simulink model "test_mdl_gw"  (R2018a)
settings: Solver=VariableStepAuto  StartTime=0.0  StopTime=10.0  RelTol=1e-3
(part 1 of 2)
settings Model: Creator=HIL105  LastModifiedBy=HIL105

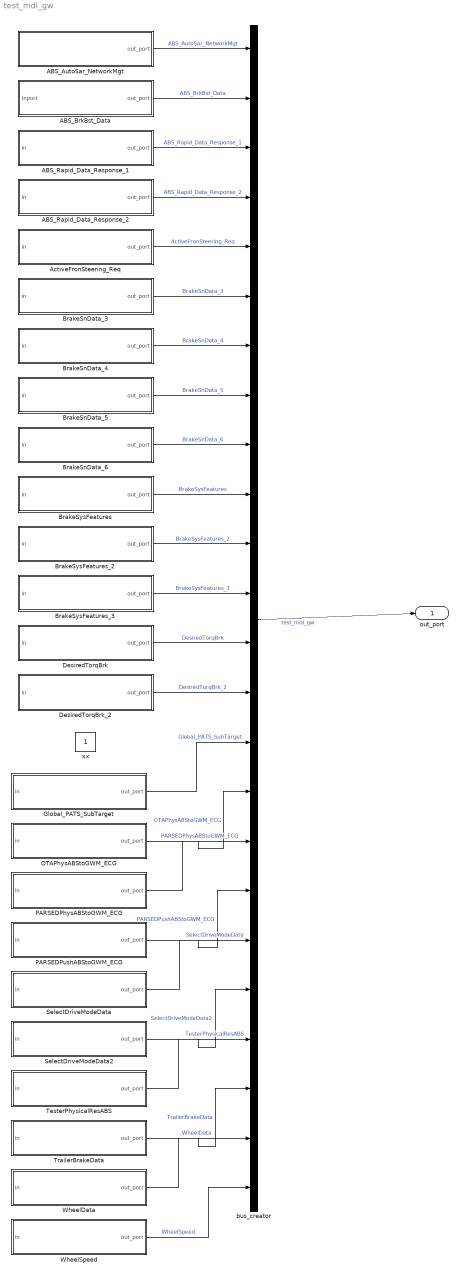
== system test_mdl_gw ==
  ABS_AutoSar_NetworkMgt : Subsystem
  ABS_BrkBst_Data : Subsystem
  ABS_Rapid_Data_Response_1 : Subsystem
  ABS_Rapid_Data_Response_2 : Subsystem
  ActiveFronSteering_Req : Subsystem
  BrakeSnData_3 : Subsystem
  BrakeSnData_4 : Subsystem
  BrakeSnData_5 : Subsystem
  BrakeSnData_6 : Subsystem
  BrakeSysFeatures : Subsystem
  BrakeSysFeatures_2 : Subsystem
  BrakeSysFeatures_3 : Subsystem
  DesiredTorqBrk : Subsystem
  DesiredTorqBrk_2 : Subsystem
  Global_PATS_SubTarget : Subsystem
  OTAPhysABStoGWM_ECG : Subsystem
  PARSEDPhysABStoGWM_ECG : Subsystem
  PARSEDPushABStoGWM_ECG : Subsystem
  SelectDriveModeData : Subsystem
  SelectDriveModeData2 : Subsystem
  TesterPhysicalResABS : Subsystem
  TrailerBrakeData : Subsystem
  WheelData : Subsystem
  WheelSpeed : Subsystem
  bus_creator : BusCreator  Inputs=24
  xx : Constant
  out_port : Outport
  wires:
  bus_creator/1 -> out_port/1  "test_mdl_gw"
  ABS_AutoSar_NetworkMgt/1(out_port) -> bus_creator/1  "ABS_AutoSar_NetworkMgt"
  ABS_BrkBst_Data/1(out_port) -> bus_creator/2  "ABS_BrkBst_Data"
  ABS_Rapid_Data_Response_1/1(out_port) -> bus_creator/3  "ABS_Rapid_Data_Response_1"
  ABS_Rapid_Data_Response_2/1(out_port) -> bus_creator/4  "ABS_Rapid_Data_Response_2"
  ActiveFronSteering_Req/1(out_port) -> bus_creator/5  "ActiveFronSteering_Req"
  BrakeSnData_3/1(out_port) -> bus_creator/6  "BrakeSnData_3"
  BrakeSnData_4/1(out_port) -> bus_creator/7  "BrakeSnData_4"
  BrakeSnData_5/1(out_port) -> bus_creator/8  "BrakeSnData_5"
  BrakeSnData_6/1(out_port) -> bus_creator/9  "BrakeSnData_6"
  BrakeSysFeatures/1(out_port) -> bus_creator/10  "BrakeSysFeatures"
  BrakeSysFeatures_2/1(out_port) -> bus_creator/11  "BrakeSysFeatures_2"
  BrakeSysFeatures_3/1(out_port) -> bus_creator/12  "BrakeSysFeatures_3"
  DesiredTorqBrk/1(out_port) -> bus_creator/13  "DesiredTorqBrk"
  DesiredTorqBrk_2/1(out_port) -> bus_creator/14  "DesiredTorqBrk_2"
  Global_PATS_SubTarget/1(out_port) -> bus_creator/15  "Global_PATS_SubTarget"
  OTAPhysABStoGWM_ECG/1(out_port) -> bus_creator/16  "OTAPhysABStoGWM_ECG"
  PARSEDPhysABStoGWM_ECG/1(out_port) -> bus_creator/17  "PARSEDPhysABStoGWM_ECG"
  PARSEDPushABStoGWM_ECG/1(out_port) -> bus_creator/18  "PARSEDPushABStoGWM_ECG"
  SelectDriveModeData/1(out_port) -> bus_creator/19  "SelectDriveModeData"
  SelectDriveModeData2/1(out_port) -> bus_creator/20  "SelectDriveModeData2"
  TesterPhysicalResABS/1(out_port) -> bus_creator/21  "TesterPhysicalResABS"
  TrailerBrakeData/1(out_port) -> bus_creator/22  "TrailerBrakeData"
  WheelData/1(out_port) -> bus_creator/23  "WheelData"
  WheelSpeed/1(out_port) -> bus_creator/24  "WheelSpeed"

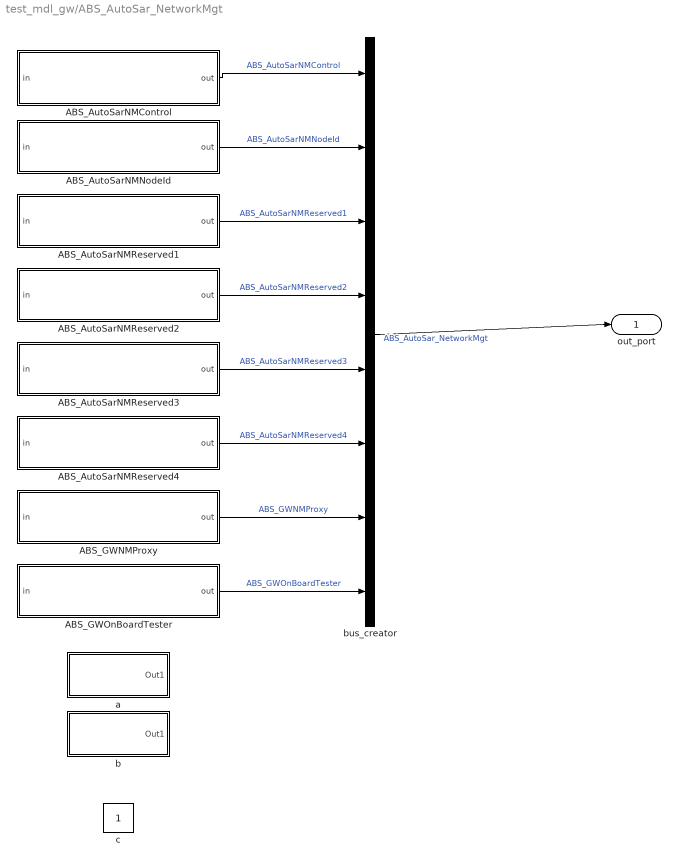
== system test_mdl_gw/ABS_AutoSar_NetworkMgt ==
  ABS_AutoSarNMControl : Subsystem
  ABS_AutoSarNMNodeId : Subsystem
  ABS_AutoSarNMReserved1 : Subsystem
  ABS_AutoSarNMReserved2 : Subsystem
  ABS_AutoSarNMReserved3 : Subsystem
  ABS_AutoSarNMReserved4 : Subsystem
  ABS_GWNMProxy : Subsystem
  ABS_GWOnBoardTester : Subsystem
  a : Subsystem
  b : Subsystem
  bus_creator : BusCreator  Inputs=8
  c : Constant
  out_port : Outport
  wires:
  bus_creator/1 -> out_port/1  "ABS_AutoSar_NetworkMgt"
  ABS_AutoSarNMControl/1(out) -> bus_creator/1  "ABS_AutoSarNMControl"
  ABS_AutoSarNMNodeId/1(out) -> bus_creator/2  "ABS_AutoSarNMNodeId"
  ABS_AutoSarNMReserved1/1(out) -> bus_creator/3  "ABS_AutoSarNMReserved1"
  ABS_AutoSarNMReserved2/1(out) -> bus_creator/4  "ABS_AutoSarNMReserved2"
  ABS_AutoSarNMReserved3/1(out) -> bus_creator/5  "ABS_AutoSarNMReserved3"
  ABS_AutoSarNMReserved4/1(out) -> bus_creator/6  "ABS_AutoSarNMReserved4"
  ABS_GWNMProxy/1(out) -> bus_creator/7  "ABS_GWNMProxy"
  ABS_GWOnBoardTester/1(out) -> bus_creator/8  "ABS_GWOnBoardTester"

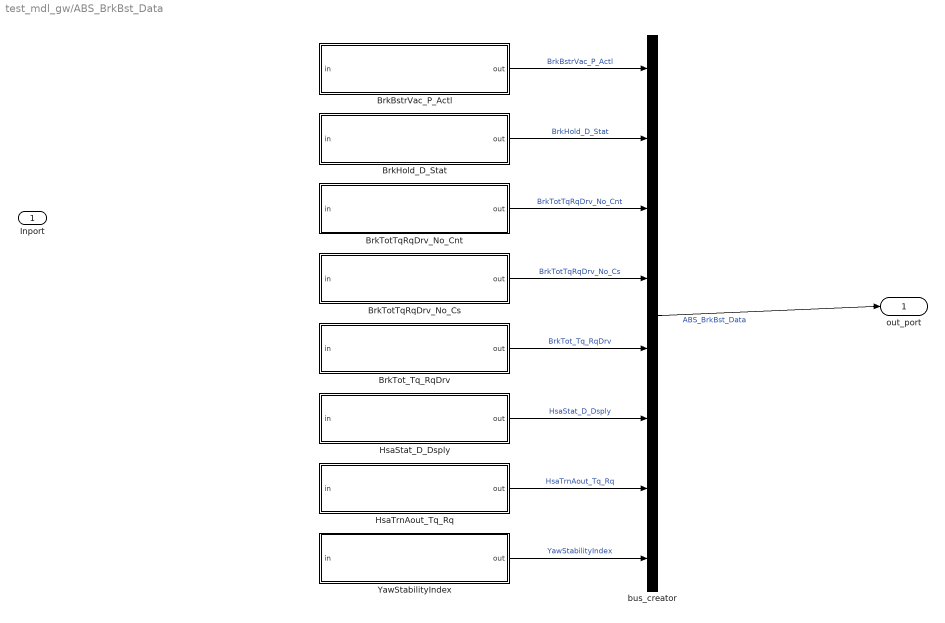
== system test_mdl_gw/ABS_BrkBst_Data ==
  Inport : Inport
  BrkBstrVac_P_Actl : Subsystem
  BrkHold_D_Stat : Subsystem
  BrkTotTqRqDrv_No_Cnt : Subsystem
  BrkTotTqRqDrv_No_Cs : Subsystem
  BrkTot_Tq_RqDrv : Subsystem
  HsaStat_D_Dsply : Subsystem
  HsaTrnAout_Tq_Rq : Subsystem
  YawStabilityIndex : Subsystem
  bus_creator : BusCreator  Inputs=8
  out_port : Outport
  wires:
  bus_creator/1 -> out_port/1  "ABS_BrkBst_Data"
  BrkBstrVac_P_Actl/1(out) -> bus_creator/1  "BrkBstrVac_P_Actl"
  BrkHold_D_Stat/1(out) -> bus_creator/2  "BrkHold_D_Stat"
  BrkTotTqRqDrv_No_Cnt/1(out) -> bus_creator/3  "BrkTotTqRqDrv_No_Cnt"
  BrkTotTqRqDrv_No_Cs/1(out) -> bus_creator/4  "BrkTotTqRqDrv_No_Cs"
  BrkTot_Tq_RqDrv/1(out) -> bus_creator/5  "BrkTot_Tq_RqDrv"
  HsaStat_D_Dsply/1(out) -> bus_creator/6  "HsaStat_D_Dsply"
  HsaTrnAout_Tq_Rq/1(out) -> bus_creator/7  "HsaTrnAout_Tq_Rq"
  YawStabilityIndex/1(out) -> bus_creator/8  "YawStabilityIndex"

== system test_mdl_gw/ABS_Rapid_Data_Response_1 ==
  in : Inport
  UUDTABSResponse1 : Subsystem
  bus_creator : BusCreator  Inputs=1
  bus_selector : BusSelector  OutputSignals=UUDTABSResponse1
  out_port : Outport
  wires:
  bus_creator/1 -> out_port/1  "ABS_Rapid_Data_Response_1"
  UUDTABSResponse1/1(out) -> bus_creator/1  "UUDTABSResponse1"
  bus_selector/1 -> UUDTABSResponse1/1(in)  "<UUDTABSResponse1>"
  in/1 -> bus_selector/1

== system test_mdl_gw/ABS_Rapid_Data_Response_2 ==
  in : Inport
  UUDTABSResponse2 : Subsystem
  bus_creator : BusCreator  Inputs=1
  bus_selector : BusSelector  OutputSignals=UUDTABSResponse2
  out_port : Outport
  wires:
  bus_creator/1 -> out_port/1  "ABS_Rapid_Data_Response_2"
  UUDTABSResponse2/1(out) -> bus_creator/1  "UUDTABSResponse2"
  bus_selector/1 -> UUDTABSResponse2/1(in)  "<UUDTABSResponse2>"
  in/1 -> bus_selector/1

== system test_mdl_gw/ActiveFronSteering_Req ==
  in : Inport
  SteWhlBrkAnRq_No_Cnt : Subsystem
  SteWhlBrkAnRq_No_Cs : Subsystem
  SteWhlBrkOffst_An_Rq : Subsystem
  bus_creator : BusCreator  Inputs=3
  bus_selector : BusSelector  OutputSignals=SteWhlBrkAnRq_No_Cnt,SteWhlBrkAnRq_No_Cs,SteWhlBrkOffst_An_Rq
  out_port : Outport
  wires:
  bus_creator/1 -> out_port/1  "ActiveFronSteering_Req"
  SteWhlBrkAnRq_No_Cnt/1(out) -> bus_creator/1  "SteWhlBrkAnRq_No_Cnt"
  SteWhlBrkAnRq_No_Cs/1(out) -> bus_creator/2  "SteWhlBrkAnRq_No_Cs"
  SteWhlBrkOffst_An_Rq/1(out) -> bus_creator/3  "SteWhlBrkOffst_An_Rq"
  bus_selector/1 -> SteWhlBrkAnRq_No_Cnt/1(in)  "<SteWhlBrkAnRq_No_Cnt>"
  bus_selector/2 -> SteWhlBrkAnRq_No_Cs/1(in)  "<SteWhlBrkAnRq_No_Cs>"
  bus_selector/3 -> SteWhlBrkOffst_An_Rq/1(in)  "<SteWhlBrkOffst_An_Rq>"
  in/1 -> bus_selector/1

== system test_mdl_gw/BrakeSnData_3 ==
  in : Inport
  VehLatComp_A_Actl : Subsystem
  VehLongComp_A_Actl : Subsystem
  VehOverGnd_V_Est : Subsystem
  VehTrvlDir_D_Stat : Subsystem
  VehYawComp_W_Actl : Subsystem
  bus_creator : BusCreator  Inputs=5
  bus_selector : BusSelector  OutputSignals=VehLatComp_A_Actl,VehLongComp_A_Actl,VehOverGnd_V_Est,VehTrvlDir_D_Stat,VehYawComp_W_Actl
  out_port : Outport
  wires:
  bus_creator/1 -> out_port/1  "BrakeSnData_3"
  VehLatComp_A_Actl/1(out) -> bus_creator/1  "VehLatComp_A_Actl"
  VehLongComp_A_Actl/1(out) -> bus_creator/2  "VehLongComp_A_Actl"
  VehOverGnd_V_Est/1(out) -> bus_creator/3  "VehOverGnd_V_Est"
  VehTrvlDir_D_Stat/1(out) -> bus_creator/4  "VehTrvlDir_D_Stat"
  VehYawComp_W_Actl/1(out) -> bus_creator/5  "VehYawComp_W_Actl"
  bus_selector/1 -> VehLatComp_A_Actl/1(in)  "<VehLatComp_A_Actl>"
  bus_selector/2 -> VehLongComp_A_Actl/1(in)  "<VehLongComp_A_Actl>"
  bus_selector/3 -> VehOverGnd_V_Est/1(in)  "<VehOverGnd_V_Est>"
  bus_selector/4 -> VehTrvlDir_D_Stat/1(in)  "<VehTrvlDir_D_Stat>"
  bus_selector/5 -> VehYawComp_W_Actl/1(in)  "<VehYawComp_W_Actl>"
  in/1 -> bus_selector/1

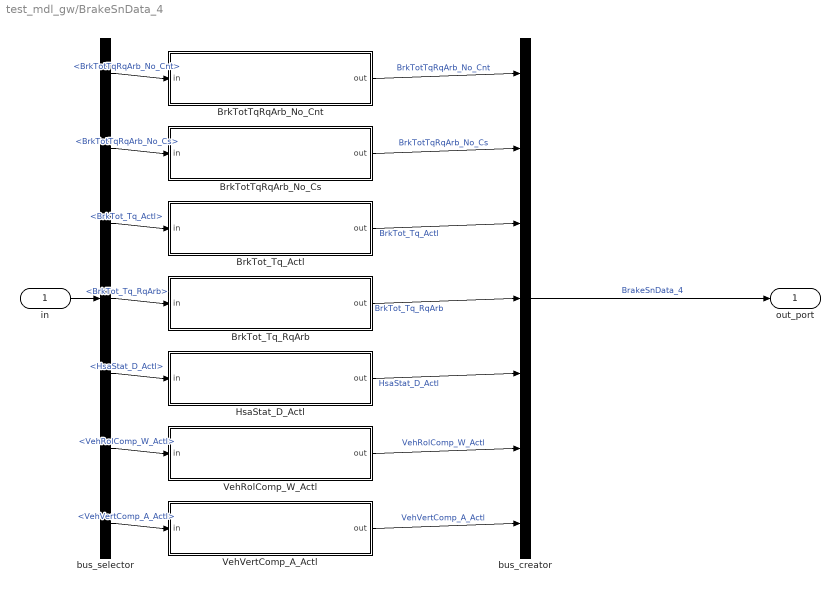
== system test_mdl_gw/BrakeSnData_4 ==
  in : Inport
  BrkTotTqRqArb_No_Cnt : Subsystem
  BrkTotTqRqArb_No_Cs : Subsystem
  BrkTot_Tq_Actl : Subsystem
  BrkTot_Tq_RqArb : Subsystem
  HsaStat_D_Actl : Subsystem
  VehRolComp_W_Actl : Subsystem
  VehVertComp_A_Actl : Subsystem
  bus_creator : BusCreator  Inputs=7
  bus_selector : BusSelector  OutputSignals=BrkTotTqRqArb_No_Cnt,BrkTotTqRqArb_No_Cs,BrkTot_Tq_Actl,BrkTot_Tq_RqArb,HsaStat_D_Actl,VehRolComp_W_Actl,VehVertComp_A_Actl
  out_port : Outport
  wires:
  bus_creator/1 -> out_port/1  "BrakeSnData_4"
  BrkTotTqRqArb_No_Cnt/1(out) -> bus_creator/1  "BrkTotTqRqArb_No_Cnt"
  BrkTotTqRqArb_No_Cs/1(out) -> bus_creator/2  "BrkTotTqRqArb_No_Cs"
  BrkTot_Tq_Actl/1(out) -> bus_creator/3  "BrkTot_Tq_Actl"
  BrkTot_Tq_RqArb/1(out) -> bus_creator/4  "BrkTot_Tq_RqArb"
  HsaStat_D_Actl/1(out) -> bus_creator/5  "HsaStat_D_Actl"
  VehRolComp_W_Actl/1(out) -> bus_creator/6  "VehRolComp_W_Actl"
  VehVertComp_A_Actl/1(out) -> bus_creator/7  "VehVertComp_A_Actl"
  bus_selector/1 -> BrkTotTqRqArb_No_Cnt/1(in)  "<BrkTotTqRqArb_No_Cnt>"
  bus_selector/2 -> BrkTotTqRqArb_No_Cs/1(in)  "<BrkTotTqRqArb_No_Cs>"
  bus_selector/3 -> BrkTot_Tq_Actl/1(in)  "<BrkTot_Tq_Actl>"
  bus_selector/4 -> BrkTot_Tq_RqArb/1(in)  "<BrkTot_Tq_RqArb>"
  bus_selector/5 -> HsaStat_D_Actl/1(in)  "<HsaStat_D_Actl>"
  bus_selector/6 -> VehRolComp_W_Actl/1(in)  "<VehRolComp_W_Actl>"
  bus_selector/7 -> VehVertComp_A_Actl/1(in)  "<VehVertComp_A_Actl>"
  in/1 -> bus_selector/1

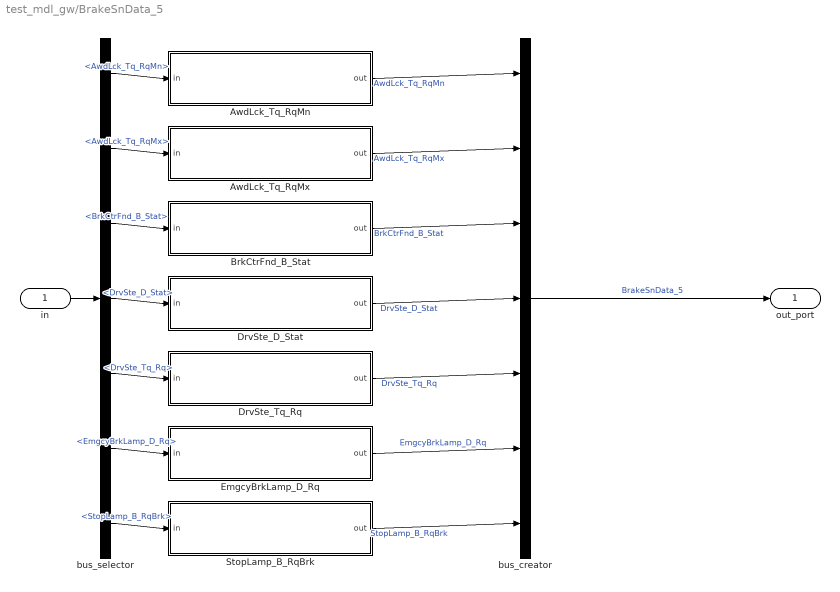
== system test_mdl_gw/BrakeSnData_5 ==
  in : Inport
  AwdLck_Tq_RqMn : Subsystem
  AwdLck_Tq_RqMx : Subsystem
  BrkCtrFnd_B_Stat : Subsystem
  DrvSte_D_Stat : Subsystem
  DrvSte_Tq_Rq : Subsystem
  EmgcyBrkLamp_D_Rq : Subsystem
  StopLamp_B_RqBrk : Subsystem
  bus_creator : BusCreator  Inputs=7
  bus_selector : BusSelector  OutputSignals=AwdLck_Tq_RqMn,AwdLck_Tq_RqMx,BrkCtrFnd_B_Stat,DrvSte_D_Stat,DrvSte_Tq_Rq,EmgcyBrkLamp_D_Rq,StopLamp_B_RqBrk
  out_port : Outport
  wires:
  bus_creator/1 -> out_port/1  "BrakeSnData_5"
  AwdLck_Tq_RqMn/1(out) -> bus_creator/1  "AwdLck_Tq_RqMn"
  AwdLck_Tq_RqMx/1(out) -> bus_creator/2  "AwdLck_Tq_RqMx"
  BrkCtrFnd_B_Stat/1(out) -> bus_creator/3  "BrkCtrFnd_B_Stat"
  DrvSte_D_Stat/1(out) -> bus_creator/4  "DrvSte_D_Stat"
  DrvSte_Tq_Rq/1(out) -> bus_creator/5  "DrvSte_Tq_Rq"
  EmgcyBrkLamp_D_Rq/1(out) -> bus_creator/6  "EmgcyBrkLamp_D_Rq"
  StopLamp_B_RqBrk/1(out) -> bus_creator/7  "StopLamp_B_RqBrk"
  bus_selector/1 -> AwdLck_Tq_RqMn/1(in)  "<AwdLck_Tq_RqMn>"
  bus_selector/2 -> AwdLck_Tq_RqMx/1(in)  "<AwdLck_Tq_RqMx>"
  bus_selector/3 -> BrkCtrFnd_B_Stat/1(in)  "<BrkCtrFnd_B_Stat>"
  bus_selector/4 -> DrvSte_D_Stat/1(in)  "<DrvSte_D_Stat>"
  bus_selector/5 -> DrvSte_Tq_Rq/1(in)  "<DrvSte_Tq_Rq>"
  bus_selector/6 -> EmgcyBrkLamp_D_Rq/1(in)  "<EmgcyBrkLamp_D_Rq>"
  bus_selector/7 -> StopLamp_B_RqBrk/1(in)  "<StopLamp_B_RqBrk>"
  in/1 -> bus_selector/1

== system test_mdl_gw/BrakeSnData_6 ==
  in : Inport
  StePinOffst_An_Est : Subsystem
  StePinOffst_D_Stat : Subsystem
  StePinOffst_No_Cnt : Subsystem
  StePinOffst_No_Cs : Subsystem
  bus_creator : BusCreator  Inputs=4
  bus_selector : BusSelector  OutputSignals=StePinOffst_An_Est,StePinOffst_D_Stat,StePinOffst_No_Cnt,StePinOffst_No_Cs
  out_port : Outport
  wires:
  bus_creator/1 -> out_port/1  "BrakeSnData_6"
  StePinOffst_An_Est/1(out) -> bus_creator/1  "StePinOffst_An_Est"
  StePinOffst_D_Stat/1(out) -> bus_creator/2  "StePinOffst_D_Stat"
  StePinOffst_No_Cnt/1(out) -> bus_creator/3  "StePinOffst_No_Cnt"
  StePinOffst_No_Cs/1(out) -> bus_creator/4  "StePinOffst_No_Cs"
  bus_selector/1 -> StePinOffst_An_Est/1(in)  "<StePinOffst_An_Est>"
  bus_selector/2 -> StePinOffst_D_Stat/1(in)  "<StePinOffst_D_Stat>"
  bus_selector/3 -> StePinOffst_No_Cnt/1(in)  "<StePinOffst_No_Cnt>"
  bus_selector/4 -> StePinOffst_No_Cs/1(in)  "<StePinOffst_No_Cs>"
  in/1 -> bus_selector/1

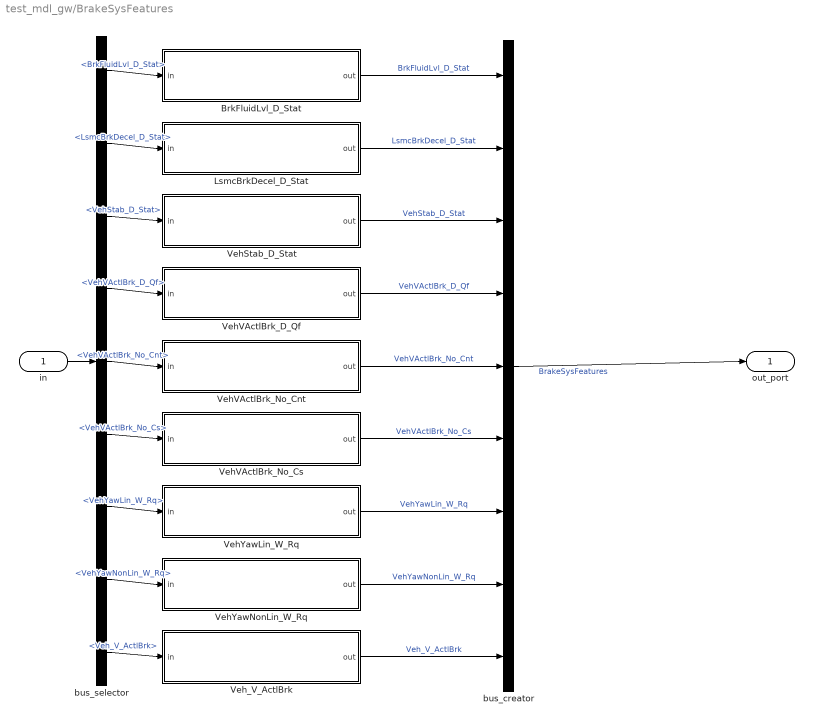
== system test_mdl_gw/BrakeSysFeatures ==
  in : Inport
  BrkFluidLvl_D_Stat : Subsystem
  LsmcBrkDecel_D_Stat : Subsystem
  VehStab_D_Stat : Subsystem
  VehVActlBrk_D_Qf : Subsystem
  VehVActlBrk_No_Cnt : Subsystem
  VehVActlBrk_No_Cs : Subsystem
  VehYawLin_W_Rq : Subsystem
  VehYawNonLin_W_Rq : Subsystem
  Veh_V_ActlBrk : Subsystem
  bus_creator : BusCreator  Inputs=9
  bus_selector : BusSelector  OutputSignals=BrkFluidLvl_D_Stat,LsmcBrkDecel_D_Stat,VehStab_D_Stat,VehVActlBrk_D_Qf,VehVActlBrk_No_Cnt,VehVActlBrk_No_Cs,VehYawLin_W_Rq,VehYawNonLin_W_Rq,Veh_V_ActlBrk
  out_port : Outport
  wires:
  bus_creator/1 -> out_port/1  "BrakeSysFeatures"
  BrkFluidLvl_D_Stat/1(out) -> bus_creator/1  "BrkFluidLvl_D_Stat"
  LsmcBrkDecel_D_Stat/1(out) -> bus_creator/2  "LsmcBrkDecel_D_Stat"
  VehStab_D_Stat/1(out) -> bus_creator/3  "VehStab_D_Stat"
  VehVActlBrk_D_Qf/1(out) -> bus_creator/4  "VehVActlBrk_D_Qf"
  VehVActlBrk_No_Cnt/1(out) -> bus_creator/5  "VehVActlBrk_No_Cnt"
  VehVActlBrk_No_Cs/1(out) -> bus_creator/6  "VehVActlBrk_No_Cs"
  VehYawLin_W_Rq/1(out) -> bus_creator/7  "VehYawLin_W_Rq"
  VehYawNonLin_W_Rq/1(out) -> bus_creator/8  "VehYawNonLin_W_Rq"
  Veh_V_ActlBrk/1(out) -> bus_creator/9  "Veh_V_ActlBrk"
  bus_selector/1 -> BrkFluidLvl_D_Stat/1(in)  "<BrkFluidLvl_D_Stat>"
  bus_selector/2 -> LsmcBrkDecel_D_Stat/1(in)  "<LsmcBrkDecel_D_Stat>"
  bus_selector/3 -> VehStab_D_Stat/1(in)  "<VehStab_D_Stat>"
  bus_selector/4 -> VehVActlBrk_D_Qf/1(in)  "<VehVActlBrk_D_Qf>"
  bus_selector/5 -> VehVActlBrk_No_Cnt/1(in)  "<VehVActlBrk_No_Cnt>"
  bus_selector/6 -> VehVActlBrk_No_Cs/1(in)  "<VehVActlBrk_No_Cs>"
  bus_selector/7 -> VehYawLin_W_Rq/1(in)  "<VehYawLin_W_Rq>"
  bus_selector/8 -> VehYawNonLin_W_Rq/1(in)  "<VehYawNonLin_W_Rq>"
  bus_selector/9 -> Veh_V_ActlBrk/1(in)  "<Veh_V_ActlBrk>"
  in/1 -> bus_selector/1

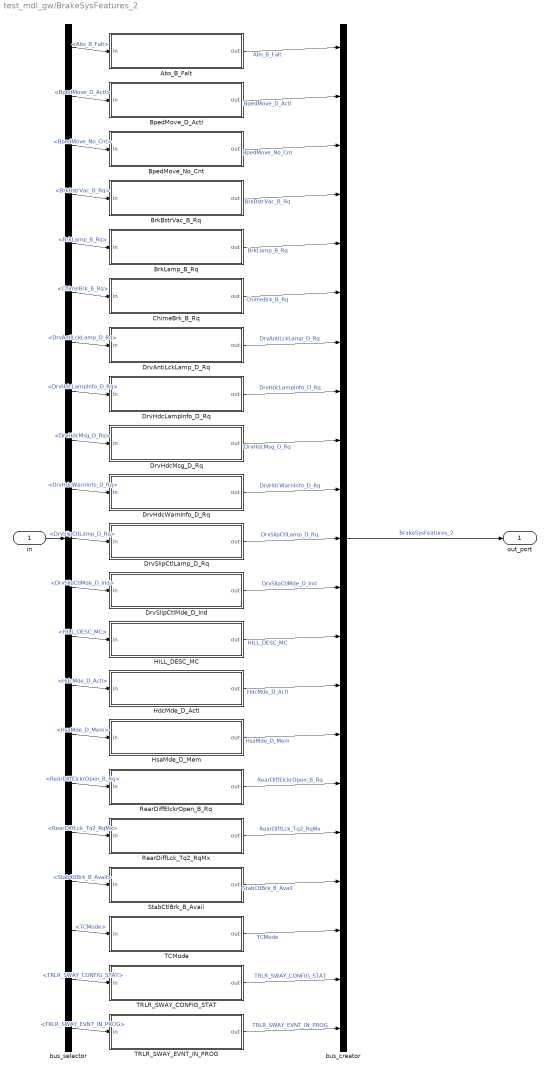
== system test_mdl_gw/BrakeSysFeatures_2 ==
  in : Inport
  Abs_B_Falt : Subsystem
  BpedMove_D_Actl : Subsystem
  BpedMove_No_Cnt : Subsystem
  BrkBstrVac_B_Rq : Subsystem
  BrkLamp_B_Rq : Subsystem
  ChimeBrk_B_Rq : Subsystem
  DrvAntiLckLamp_D_Rq : Subsystem
  DrvHdcLampInfo_D_Rq : Subsystem
  DrvHdcMsg_D_Rq : Subsystem
  DrvHdcWarnInfo_D_Rq : Subsystem
  DrvSlipCtlLamp_D_Rq : Subsystem
  DrvSlipCtlMde_D_Ind : Subsystem
  HILL_DESC_MC : Subsystem
  HdcMde_D_Actl : Subsystem
  HsaMde_D_Mem : Subsystem
  RearDiffElckrOpen_B_Rq : Subsystem
  RearDiffLck_Tq2_RqMx : Subsystem
  StabCtlBrk_B_Avail : Subsystem
  TCMode : Subsystem
  TRLR_SWAY_CONFIG_STAT : Subsystem
  TRLR_SWAY_EVNT_IN_PROG : Subsystem
  bus_creator : BusCreator  Inputs=21
  bus_selector : BusSelector  OutputSignals=Abs_B_Falt,BpedMove_D_Actl,BpedMove_No_Cnt,BrkBstrVac_B_Rq,BrkLamp_B_Rq,ChimeBrk_B_Rq,DrvAntiLckLamp_D_Rq,DrvHdcLampInfo_D_Rq,DrvHdcMsg_D_Rq,DrvHdcWarnInfo_D_Rq,DrvSlipCtlLamp_D_Rq,DrvSlipCtlMde_D_Ind,HILL_DESC_MC,HdcMde_D_Actl,HsaMde_D_Mem,RearDiffElckrOpen_B_Rq,RearDiffLck_Tq2_RqMx,StabCtlBrk_B_Avail,TCMode,TRLR_SWAY_CONFIG_STAT,TRLR_SWAY_EVNT_IN_PROG
  out_port : Outport
  wires:
  bus_creator/1 -> out_port/1  "BrakeSysFeatures_2"
  Abs_B_Falt/1(out) -> bus_creator/1  "Abs_B_Falt"
  BpedMove_D_Actl/1(out) -> bus_creator/2  "BpedMove_D_Actl"
  BpedMove_No_Cnt/1(out) -> bus_creator/3  "BpedMove_No_Cnt"
  BrkBstrVac_B_Rq/1(out) -> bus_creator/4  "BrkBstrVac_B_Rq"
  BrkLamp_B_Rq/1(out) -> bus_creator/5  "BrkLamp_B_Rq"
  ChimeBrk_B_Rq/1(out) -> bus_creator/6  "ChimeBrk_B_Rq"
  DrvAntiLckLamp_D_Rq/1(out) -> bus_creator/7  "DrvAntiLckLamp_D_Rq"
  DrvHdcLampInfo_D_Rq/1(out) -> bus_creator/8  "DrvHdcLampInfo_D_Rq"
  DrvHdcMsg_D_Rq/1(out) -> bus_creator/9  "DrvHdcMsg_D_Rq"
  DrvHdcWarnInfo_D_Rq/1(out) -> bus_creator/10  "DrvHdcWarnInfo_D_Rq"
  DrvSlipCtlLamp_D_Rq/1(out) -> bus_creator/11  "DrvSlipCtlLamp_D_Rq"
  DrvSlipCtlMde_D_Ind/1(out) -> bus_creator/12  "DrvSlipCtlMde_D_Ind"
  HILL_DESC_MC/1(out) -> bus_creator/13  "HILL_DESC_MC"
  HdcMde_D_Actl/1(out) -> bus_creator/14  "HdcMde_D_Actl"
  HsaMde_D_Mem/1(out) -> bus_creator/15  "HsaMde_D_Mem"
  RearDiffElckrOpen_B_Rq/1(out) -> bus_creator/16  "RearDiffElckrOpen_B_Rq"
  RearDiffLck_Tq2_RqMx/1(out) -> bus_creator/17  "RearDiffLck_Tq2_RqMx"
  StabCtlBrk_B_Avail/1(out) -> bus_creator/18  "StabCtlBrk_B_Avail"
  TCMode/1(out) -> bus_creator/19  "TCMode"
  TRLR_SWAY_CONFIG_STAT/1(out) -> bus_creator/20  "TRLR_SWAY_CONFIG_STAT"
  TRLR_SWAY_EVNT_IN_PROG/1(out) -> bus_creator/21  "TRLR_SWAY_EVNT_IN_PROG"
  bus_selector/1 -> Abs_B_Falt/1(in)  "<Abs_B_Falt>"
  bus_selector/2 -> BpedMove_D_Actl/1(in)  "<BpedMove_D_Actl>"
  bus_selector/3 -> BpedMove_No_Cnt/1(in)  "<BpedMove_No_Cnt>"
  bus_selector/4 -> BrkBstrVac_B_Rq/1(in)  "<BrkBstrVac_B_Rq>"
  bus_selector/5 -> BrkLamp_B_Rq/1(in)  "<BrkLamp_B_Rq>"
  bus_selector/6 -> ChimeBrk_B_Rq/1(in)  "<ChimeBrk_B_Rq>"
  bus_selector/7 -> DrvAntiLckLamp_D_Rq/1(in)  "<DrvAntiLckLamp_D_Rq>"
  bus_selector/8 -> DrvHdcLampInfo_D_Rq/1(in)  "<DrvHdcLampInfo_D_Rq>"
  bus_selector/9 -> DrvHdcMsg_D_Rq/1(in)  "<DrvHdcMsg_D_Rq>"
  bus_selector/10 -> DrvHdcWarnInfo_D_Rq/1(in)  "<DrvHdcWarnInfo_D_Rq>"
  bus_selector/11 -> DrvSlipCtlLamp_D_Rq/1(in)  "<DrvSlipCtlLamp_D_Rq>"
  bus_selector/12 -> DrvSlipCtlMde_D_Ind/1(in)  "<DrvSlipCtlMde_D_Ind>"
  bus_selector/13 -> HILL_DESC_MC/1(in)  "<HILL_DESC_MC>"
  bus_selector/14 -> HdcMde_D_Actl/1(in)  "<HdcMde_D_Actl>"
  bus_selector/15 -> HsaMde_D_Mem/1(in)  "<HsaMde_D_Mem>"
  bus_selector/16 -> RearDiffElckrOpen_B_Rq/1(in)  "<RearDiffElckrOpen_B_Rq>"
  bus_selector/17 -> RearDiffLck_Tq2_RqMx/1(in)  "<RearDiffLck_Tq2_RqMx>"
  bus_selector/18 -> StabCtlBrk_B_Avail/1(in)  "<StabCtlBrk_B_Avail>"
  bus_selector/19 -> TCMode/1(in)  "<TCMode>"
  bus_selector/20 -> TRLR_SWAY_CONFIG_STAT/1(in)  "<TRLR_SWAY_CONFIG_STAT>"
  bus_selector/21 -> TRLR_SWAY_EVNT_IN_PROG/1(in)  "<TRLR_SWAY_EVNT_IN_PROG>"
  in/1 -> bus_selector/1

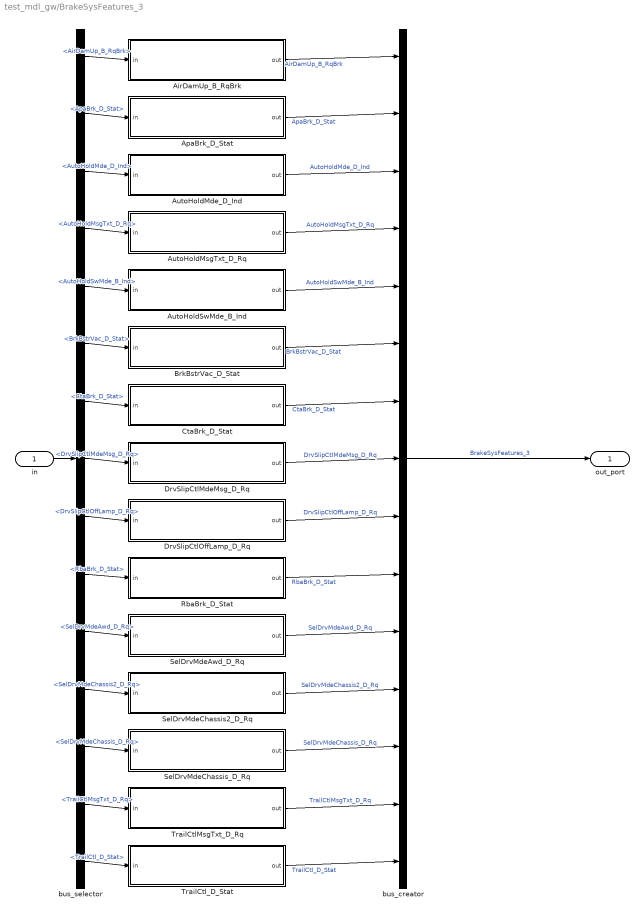
== system test_mdl_gw/BrakeSysFeatures_3 ==
  in : Inport
  AirDamUp_B_RqBrk : Subsystem
  ApaBrk_D_Stat : Subsystem
  AutoHoldMde_D_Ind : Subsystem
  AutoHoldMsgTxt_D_Rq : Subsystem
  AutoHoldSwMde_B_Ind : Subsystem
  BrkBstrVac_D_Stat : Subsystem
  CtaBrk_D_Stat : Subsystem
  DrvSlipCtlMdeMsg_D_Rq : Subsystem
  DrvSlipCtlOffLamp_D_Rq : Subsystem
  RbaBrk_D_Stat : Subsystem
  SelDrvMdeAwd_D_Rq : Subsystem
  SelDrvMdeChassis2_D_Rq : Subsystem
  SelDrvMdeChassis_D_Rq : Subsystem
  TrailCtlMsgTxt_D_Rq : Subsystem
  TrailCtl_D_Stat : Subsystem
  bus_creator : BusCreator  Inputs=15
  bus_selector : BusSelector  OutputSignals=AirDamUp_B_RqBrk,ApaBrk_D_Stat,AutoHoldMde_D_Ind,AutoHoldMsgTxt_D_Rq,AutoHoldSwMde_B_Ind,BrkBstrVac_D_Stat,CtaBrk_D_Stat,DrvSlipCtlMdeMsg_D_Rq,DrvSlipCtlOffLamp_D_Rq,RbaBrk_D_Stat,SelDrvMdeAwd_D_Rq,SelDrvMdeChassis2_D_Rq,SelDrvMdeChassis_D_Rq,TrailCtlMsgTxt_D_Rq,TrailCtl_D_Stat
  out_port : Outport
  wires:
  bus_creator/1 -> out_port/1  "BrakeSysFeatures_3"
  AirDamUp_B_RqBrk/1(out) -> bus_creator/1  "AirDamUp_B_RqBrk"
  ApaBrk_D_Stat/1(out) -> bus_creator/2  "ApaBrk_D_Stat"
  AutoHoldMde_D_Ind/1(out) -> bus_creator/3  "AutoHoldMde_D_Ind"
  AutoHoldMsgTxt_D_Rq/1(out) -> bus_creator/4  "AutoHoldMsgTxt_D_Rq"
  AutoHoldSwMde_B_Ind/1(out) -> bus_creator/5  "AutoHoldSwMde_B_Ind"
  BrkBstrVac_D_Stat/1(out) -> bus_creator/6  "BrkBstrVac_D_Stat"
  CtaBrk_D_Stat/1(out) -> bus_creator/7  "CtaBrk_D_Stat"
  DrvSlipCtlMdeMsg_D_Rq/1(out) -> bus_creator/8  "DrvSlipCtlMdeMsg_D_Rq"
  DrvSlipCtlOffLamp_D_Rq/1(out) -> bus_creator/9  "DrvSlipCtlOffLamp_D_Rq"
  RbaBrk_D_Stat/1(out) -> bus_creator/10  "RbaBrk_D_Stat"
  SelDrvMdeAwd_D_Rq/1(out) -> bus_creator/11  "SelDrvMdeAwd_D_Rq"
  SelDrvMdeChassis2_D_Rq/1(out) -> bus_creator/12  "SelDrvMdeChassis2_D_Rq"
  SelDrvMdeChassis_D_Rq/1(out) -> bus_creator/13  "SelDrvMdeChassis_D_Rq"
  TrailCtlMsgTxt_D_Rq/1(out) -> bus_creator/14  "TrailCtlMsgTxt_D_Rq"
  TrailCtl_D_Stat/1(out) -> bus_creator/15  "TrailCtl_D_Stat"
  bus_selector/1 -> AirDamUp_B_RqBrk/1(in)  "<AirDamUp_B_RqBrk>"
  bus_selector/2 -> ApaBrk_D_Stat/1(in)  "<ApaBrk_D_Stat>"
  bus_selector/3 -> AutoHoldMde_D_Ind/1(in)  "<AutoHoldMde_D_Ind>"
  bus_selector/4 -> AutoHoldMsgTxt_D_Rq/1(in)  "<AutoHoldMsgTxt_D_Rq>"
  bus_selector/5 -> AutoHoldSwMde_B_Ind/1(in)  "<AutoHoldSwMde_B_Ind>"
  bus_selector/6 -> BrkBstrVac_D_Stat/1(in)  "<BrkBstrVac_D_Stat>"
  bus_selector/7 -> CtaBrk_D_Stat/1(in)  "<CtaBrk_D_Stat>"
  bus_selector/8 -> DrvSlipCtlMdeMsg_D_Rq/1(in)  "<DrvSlipCtlMdeMsg_D_Rq>"
  bus_selector/9 -> DrvSlipCtlOffLamp_D_Rq/1(in)  "<DrvSlipCtlOffLamp_D_Rq>"
  bus_selector/10 -> RbaBrk_D_Stat/1(in)  "<RbaBrk_D_Stat>"
  bus_selector/11 -> SelDrvMdeAwd_D_Rq/1(in)  "<SelDrvMdeAwd_D_Rq>"
  bus_selector/12 -> SelDrvMdeChassis2_D_Rq/1(in)  "<SelDrvMdeChassis2_D_Rq>"
  bus_selector/13 -> SelDrvMdeChassis_D_Rq/1(in)  "<SelDrvMdeChassis_D_Rq>"
  bus_selector/14 -> TrailCtlMsgTxt_D_Rq/1(in)  "<TrailCtlMsgTxt_D_Rq>"
  bus_selector/15 -> TrailCtl_D_Stat/1(in)  "<TrailCtl_D_Stat>"
  in/1 -> bus_selector/1

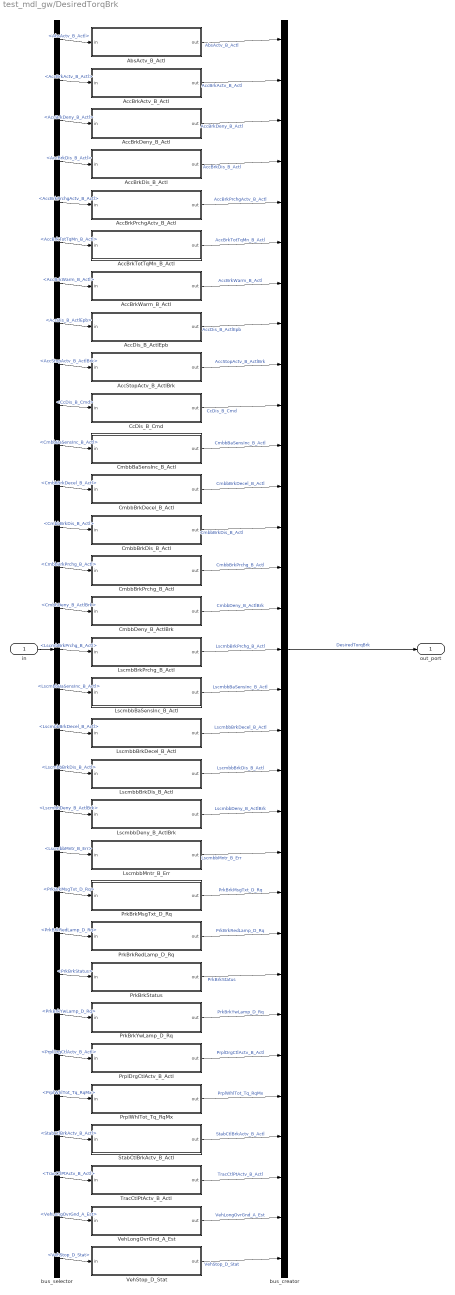
== system test_mdl_gw/DesiredTorqBrk ==
  in : Inport
  AbsActv_B_Actl : Subsystem
  AccBrkActv_B_Actl : Subsystem
  AccBrkDeny_B_Actl : Subsystem
  AccBrkDis_B_Actl : Subsystem
  AccBrkPrchgActv_B_Actl : Subsystem
  AccBrkTotTqMn_B_Actl : Subsystem
  AccBrkWarm_B_Actl : Subsystem
  AccDis_B_ActlEpb : Subsystem
  AccStopActv_B_ActlBrk : Subsystem
  CcDis_B_Cmd : Subsystem
  CmbbBaSensInc_B_Actl : Subsystem
  CmbbBrkDecel_B_Actl : Subsystem
  CmbbBrkDis_B_Actl : Subsystem
  CmbbBrkPrchg_B_Actl : Subsystem
  CmbbDeny_B_ActlBrk : Subsystem
  LscmbBrkPrchg_B_Actl : Subsystem
  LscmbbBaSensInc_B_Actl : Subsystem
  LscmbbBrkDecel_B_Actl : Subsystem
  LscmbbBrkDis_B_Actl : Subsystem
  LscmbbDeny_B_ActlBrk : Subsystem
  LscmbbMntr_B_Err : Subsystem
  PrkBrkMsgTxt_D_Rq : Subsystem
  PrkBrkRedLamp_D_Rq : Subsystem
  PrkBrkStatus : Subsystem
  PrkBrkYwLamp_D_Rq : Subsystem
  PrplDrgCtlActv_B_Actl : Subsystem
  PrplWhlTot_Tq_RqMx : Subsystem
  StabCtlBrkActv_B_Actl : Subsystem
  TracCtlPtActv_B_Actl : Subsystem
  VehLongOvrGnd_A_Est : Subsystem
  VehStop_D_Stat : Subsystem
  bus_creator : BusCreator  Inputs=31
  bus_selector : BusSelector  OutputSignals=AbsActv_B_Actl,AccBrkActv_B_Actl,AccBrkDeny_B_Actl,AccBrkDis_B_Actl,AccBrkPrchgActv_B_Actl,AccBrkTotTqMn_B_Actl,AccBrkWarm_B_Actl,AccDis_B_ActlEpb,AccStopActv_B_ActlBrk,CcDis_B_Cmd,CmbbBaSensInc_B_Actl,CmbbBrkDecel_B_Actl,CmbbBrkDis_B_Actl,CmbbBrkPrchg_B_Actl,CmbbDeny_B_ActlBrk,LscmbBrkPrchg_B_Actl,LscmbbBaSensInc_B_Actl,LscmbbBrkDecel_B_Actl,LscmbbBrkDis_B_Actl,LscmbbDeny_B_ActlBrk,LscmbbMntr_B_Err,PrkBrkMsgTxt_D_Rq,PrkBrkRedLamp_D_Rq,PrkBrkStatus,PrkBrkYwLamp_D_Rq,PrplDrgCtlActv_B_Actl,PrplWhlTot_Tq_RqMx,StabCtlBrkActv_B_Actl,TracCtlPtActv_B_Actl,VehLongOvrGnd_A_Est,VehStop_D_Stat
  out_port : Outport
  wires:
  bus_creator/1 -> out_port/1  "DesiredTorqBrk"
  AbsActv_B_Actl/1(out) -> bus_creator/1  "AbsActv_B_Actl"
  AccBrkActv_B_Actl/1(out) -> bus_creator/2  "AccBrkActv_B_Actl"
  AccBrkDeny_B_Actl/1(out) -> bus_creator/3  "AccBrkDeny_B_Actl"
  AccBrkDis_B_Actl/1(out) -> bus_creator/4  "AccBrkDis_B_Actl"
  AccBrkPrchgActv_B_Actl/1(out) -> bus_creator/5  "AccBrkPrchgActv_B_Actl"
  AccBrkTotTqMn_B_Actl/1(out) -> bus_creator/6  "AccBrkTotTqMn_B_Actl"
  AccBrkWarm_B_Actl/1(out) -> bus_creator/7  "AccBrkWarm_B_Actl"
  AccDis_B_ActlEpb/1(out) -> bus_creator/8  "AccDis_B_ActlEpb"
  AccStopActv_B_ActlBrk/1(out) -> bus_creator/9  "AccStopActv_B_ActlBrk"
  CcDis_B_Cmd/1(out) -> bus_creator/10  "CcDis_B_Cmd"
  CmbbBaSensInc_B_Actl/1(out) -> bus_creator/11  "CmbbBaSensInc_B_Actl"
  CmbbBrkDecel_B_Actl/1(out) -> bus_creator/12  "CmbbBrkDecel_B_Actl"
  CmbbBrkDis_B_Actl/1(out) -> bus_creator/13  "CmbbBrkDis_B_Actl"
  CmbbBrkPrchg_B_Actl/1(out) -> bus_creator/14  "CmbbBrkPrchg_B_Actl"
  CmbbDeny_B_ActlBrk/1(out) -> bus_creator/15  "CmbbDeny_B_ActlBrk"
  LscmbBrkPrchg_B_Actl/1(out) -> bus_creator/16  "LscmbBrkPrchg_B_Actl"
  LscmbbBaSensInc_B_Actl/1(out) -> bus_creator/17  "LscmbbBaSensInc_B_Actl"
  LscmbbBrkDecel_B_Actl/1(out) -> bus_creator/18  "LscmbbBrkDecel_B_Actl"
  LscmbbBrkDis_B_Actl/1(out) -> bus_creator/19  "LscmbbBrkDis_B_Actl"
  LscmbbDeny_B_ActlBrk/1(out) -> bus_creator/20  "LscmbbDeny_B_ActlBrk"
  LscmbbMntr_B_Err/1(out) -> bus_creator/21  "LscmbbMntr_B_Err"
  PrkBrkMsgTxt_D_Rq/1(out) -> bus_creator/22  "PrkBrkMsgTxt_D_Rq"
  PrkBrkRedLamp_D_Rq/1(out) -> bus_creator/23  "PrkBrkRedLamp_D_Rq"
  PrkBrkStatus/1(out) -> bus_creator/24  "PrkBrkStatus"
  PrkBrkYwLamp_D_Rq/1(out) -> bus_creator/25  "PrkBrkYwLamp_D_Rq"
  PrplDrgCtlActv_B_Actl/1(out) -> bus_creator/26  "PrplDrgCtlActv_B_Actl"
  PrplWhlTot_Tq_RqMx/1(out) -> bus_creator/27  "PrplWhlTot_Tq_RqMx"
  StabCtlBrkActv_B_Actl/1(out) -> bus_creator/28  "StabCtlBrkActv_B_Actl"
  TracCtlPtActv_B_Actl/1(out) -> bus_creator/29  "TracCtlPtActv_B_Actl"
  VehLongOvrGnd_A_Est/1(out) -> bus_creator/30  "VehLongOvrGnd_A_Est"
  VehStop_D_Stat/1(out) -> bus_creator/31  "VehStop_D_Stat"
  bus_selector/1 -> AbsActv_B_Actl/1(in)  "<AbsActv_B_Actl>"
  bus_selector/2 -> AccBrkActv_B_Actl/1(in)  "<AccBrkActv_B_Actl>"
  bus_selector/3 -> AccBrkDeny_B_Actl/1(in)  "<AccBrkDeny_B_Actl>"
  bus_selector/4 -> AccBrkDis_B_Actl/1(in)  "<AccBrkDis_B_Actl>"
  bus_selector/5 -> AccBrkPrchgActv_B_Actl/1(in)  "<AccBrkPrchgActv_B_Actl>"
  bus_selector/6 -> AccBrkTotTqMn_B_Actl/1(in)  "<AccBrkTotTqMn_B_Actl>"
  bus_selector/7 -> AccBrkWarm_B_Actl/1(in)  "<AccBrkWarm_B_Actl>"
  bus_selector/8 -> AccDis_B_ActlEpb/1(in)  "<AccDis_B_ActlEpb>"
  bus_selector/9 -> AccStopActv_B_ActlBrk/1(in)  "<AccStopActv_B_ActlBrk>"
  bus_selector/10 -> CcDis_B_Cmd/1(in)  "<CcDis_B_Cmd>"
  bus_selector/11 -> CmbbBaSensInc_B_Actl/1(in)  "<CmbbBaSensInc_B_Actl>"
  bus_selector/12 -> CmbbBrkDecel_B_Actl/1(in)  "<CmbbBrkDecel_B_Actl>"
  bus_selector/13 -> CmbbBrkDis_B_Actl/1(in)  "<CmbbBrkDis_B_Actl>"
  bus_selector/14 -> CmbbBrkPrchg_B_Actl/1(in)  "<CmbbBrkPrchg_B_Actl>"
  bus_selector/15 -> CmbbDeny_B_ActlBrk/1(in)  "<CmbbDeny_B_ActlBrk>"
  bus_selector/16 -> LscmbBrkPrchg_B_Actl/1(in)  "<LscmbBrkPrchg_B_Actl>"
  bus_selector/17 -> LscmbbBaSensInc_B_Actl/1(in)  "<LscmbbBaSensInc_B_Actl>"
  bus_selector/18 -> LscmbbBrkDecel_B_Actl/1(in)  "<LscmbbBrkDecel_B_Actl>"
  bus_selector/19 -> LscmbbBrkDis_B_Actl/1(in)  "<LscmbbBrkDis_B_Actl>"
  bus_selector/20 -> LscmbbDeny_B_ActlBrk/1(in)  "<LscmbbDeny_B_ActlBrk>"
  bus_selector/21 -> LscmbbMntr_B_Err/1(in)  "<LscmbbMntr_B_Err>"
  bus_selector/22 -> PrkBrkMsgTxt_D_Rq/1(in)  "<PrkBrkMsgTxt_D_Rq>"
  bus_selector/23 -> PrkBrkRedLamp_D_Rq/1(in)  "<PrkBrkRedLamp_D_Rq>"
  bus_selector/24 -> PrkBrkStatus/1(in)  "<PrkBrkStatus>"
  bus_selector/25 -> PrkBrkYwLamp_D_Rq/1(in)  "<PrkBrkYwLamp_D_Rq>"
  bus_selector/26 -> PrplDrgCtlActv_B_Actl/1(in)  "<PrplDrgCtlActv_B_Actl>"
  bus_selector/27 -> PrplWhlTot_Tq_RqMx/1(in)  "<PrplWhlTot_Tq_RqMx>"
  bus_selector/28 -> StabCtlBrkActv_B_Actl/1(in)  "<StabCtlBrkActv_B_Actl>"
  bus_selector/29 -> TracCtlPtActv_B_Actl/1(in)  "<TracCtlPtActv_B_Actl>"
  bus_selector/30 -> VehLongOvrGnd_A_Est/1(in)  "<VehLongOvrGnd_A_Est>"
  bus_selector/31 -> VehStop_D_Stat/1(in)  "<VehStop_D_Stat>"
  in/1 -> bus_selector/1

== system test_mdl_gw/DesiredTorqBrk_2 ==
  in : Inport
  PrplWhlTot_Tq_RqMn : Subsystem
  PrplWhlTqRqMn_No_Cnt : Subsystem
  PrplWhlTqRqMn_No_Cs : Subsystem
  RgenBrkDynoMde_B_Actl : Subsystem
  RgenTqFalt_B_Actl : Subsystem
  bus_creator : BusCreator  Inputs=5
  bus_selector : BusSelector  OutputSignals=PrplWhlTot_Tq_RqMn,PrplWhlTqRqMn_No_Cnt,PrplWhlTqRqMn_No_Cs,RgenBrkDynoMde_B_Actl,RgenTqFalt_B_Actl
  out_port : Outport
  wires:
  bus_creator/1 -> out_port/1  "DesiredTorqBrk_2"
  PrplWhlTot_Tq_RqMn/1(out) -> bus_creator/1  "PrplWhlTot_Tq_RqMn"
  PrplWhlTqRqMn_No_Cnt/1(out) -> bus_creator/2  "PrplWhlTqRqMn_No_Cnt"
  PrplWhlTqRqMn_No_Cs/1(out) -> bus_creator/3  "PrplWhlTqRqMn_No_Cs"
  RgenBrkDynoMde_B_Actl/1(out) -> bus_creator/4  "RgenBrkDynoMde_B_Actl"
  RgenTqFalt_B_Actl/1(out) -> bus_creator/5  "RgenTqFalt_B_Actl"
  bus_selector/1 -> PrplWhlTot_Tq_RqMn/1(in)  "<PrplWhlTot_Tq_RqMn>"
  bus_selector/2 -> PrplWhlTqRqMn_No_Cnt/1(in)  "<PrplWhlTqRqMn_No_Cnt>"
  bus_selector/3 -> PrplWhlTqRqMn_No_Cs/1(in)  "<PrplWhlTqRqMn_No_Cs>"
  bus_selector/4 -> RgenBrkDynoMde_B_Actl/1(in)  "<RgenBrkDynoMde_B_Actl>"
  bus_selector/5 -> RgenTqFalt_B_Actl/1(in)  "<RgenTqFalt_B_Actl>"
  in/1 -> bus_selector/1

== system test_mdl_gw/Global_PATS_SubTarget ==
  in : Inport
  bus_creator : BusCreator  Inputs=2
  bus_selector : BusSelector  OutputSignals=immoSubTarget1Cmd_T1,immoSubTarget1Data_T1
  immoSubTarget1Cmd_T1 : Subsystem
  immoSubTarget1Data_T1 : Subsystem
  out_port : Outport
  wires:
  bus_creator/1 -> out_port/1  "Global_PATS_SubTarget"
  immoSubTarget1Cmd_T1/1(out) -> bus_creator/1  "immoSubTarget1Cmd_T1"
  immoSubTarget1Data_T1/1(out) -> bus_creator/2  "immoSubTarget1Data_T1"
  bus_selector/1 -> immoSubTarget1Cmd_T1/1(in)  "<immoSubTarget1Cmd_T1>"
  bus_selector/2 -> immoSubTarget1Data_T1/1(in)  "<immoSubTarget1Data_T1>"
  in/1 -> bus_selector/1

== system test_mdl_gw/OTAPhysABStoGWM_ECG ==
  in : Inport
  OTAPhysABStoGWM_ECG : Subsystem
  bus_creator : BusCreator  Inputs=1
  bus_selector : BusSelector  OutputSignals=OTAPhysABStoGWM_ECG
  out_port : Outport
  wires:
  bus_creator/1 -> out_port/1  "OTAPhysABStoGWM_ECG"
  OTAPhysABStoGWM_ECG/1(out) -> bus_creator/1  "OTAPhysABStoGWM_ECG"
  bus_selector/1 -> OTAPhysABStoGWM_ECG/1(in)  "<OTAPhysABStoGWM_ECG>"
  in/1 -> bus_selector/1

== system test_mdl_gw/PARSEDPhysABStoGWM_ECG ==
  in : Inport
  PARSEDPhysABStoGWM_ECG : Subsystem
  bus_creator : BusCreator  Inputs=1
  bus_selector : BusSelector  OutputSignals=PARSEDPhysABStoGWM_ECG
  out_port : Outport
  wires:
  bus_creator/1 -> out_port/1  "PARSEDPhysABStoGWM_ECG"
  PARSEDPhysABStoGWM_ECG/1(out) -> bus_creator/1  "PARSEDPhysABStoGWM_ECG"
  bus_selector/1 -> PARSEDPhysABStoGWM_ECG/1(in)  "<PARSEDPhysABStoGWM_ECG>"
  in/1 -> bus_selector/1

== system test_mdl_gw/PARSEDPushABStoGWM_ECG ==
  in : Inport
  PARSEDPhysABS2toGWM_ECG : Subsystem
  bus_creator : BusCreator  Inputs=1
  bus_selector : BusSelector  OutputSignals=PARSEDPhysABS2toGWM_ECG
  out_port : Outport
  wires:
  bus_creator/1 -> out_port/1  "PARSEDPushABStoGWM_ECG"
  PARSEDPhysABS2toGWM_ECG/1(out) -> bus_creator/1  "PARSEDPhysABS2toGWM_ECG"
  bus_selector/1 -> PARSEDPhysABS2toGWM_ECG/1(in)  "<PARSEDPhysABS2toGWM_ECG>"
  in/1 -> bus_selector/1

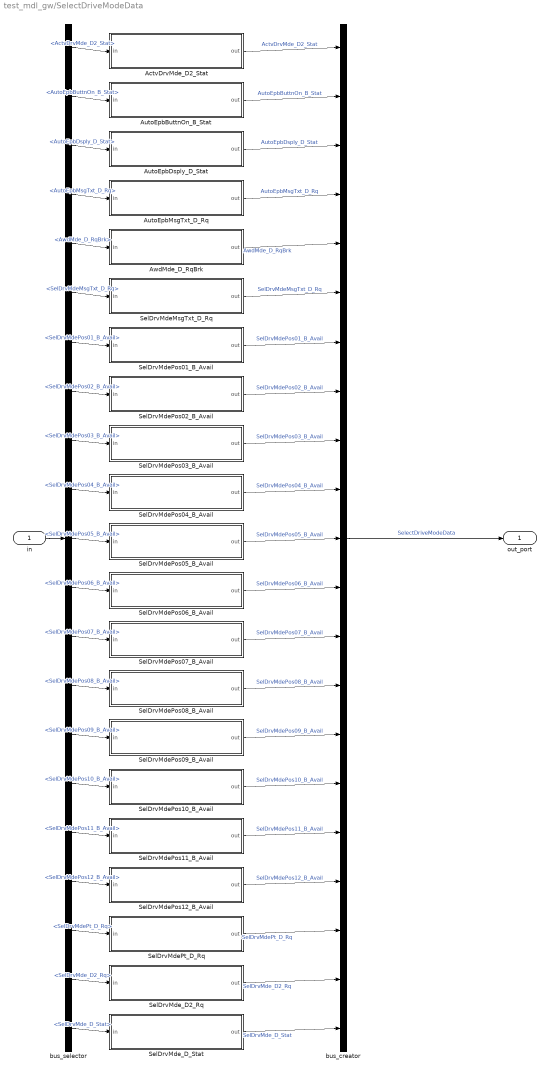
== system test_mdl_gw/SelectDriveModeData ==
  in : Inport
  ActvDrvMde_D2_Stat : Subsystem
  AutoEpbButtnOn_B_Stat : Subsystem
  AutoEpbDsply_D_Stat : Subsystem
  AutoEpbMsgTxt_D_Rq : Subsystem
  AwdMde_D_RqBrk : Subsystem
  SelDrvMdeMsgTxt_D_Rq : Subsystem
  SelDrvMdePos01_B_Avail : Subsystem
  SelDrvMdePos02_B_Avail : Subsystem
  SelDrvMdePos03_B_Avail : Subsystem
  SelDrvMdePos04_B_Avail : Subsystem
  SelDrvMdePos05_B_Avail : Subsystem
  SelDrvMdePos06_B_Avail : Subsystem
  SelDrvMdePos07_B_Avail : Subsystem
  SelDrvMdePos08_B_Avail : Subsystem
  SelDrvMdePos09_B_Avail : Subsystem
  SelDrvMdePos10_B_Avail : Subsystem
  SelDrvMdePos11_B_Avail : Subsystem
  SelDrvMdePos12_B_Avail : Subsystem
  SelDrvMdePt_D_Rq : Subsystem
  SelDrvMde_D2_Rq : Subsystem
  SelDrvMde_D_Stat : Subsystem
  bus_creator : BusCreator  Inputs=21
  bus_selector : BusSelector  OutputSignals=ActvDrvMde_D2_Stat,AutoEpbButtnOn_B_Stat,AutoEpbDsply_D_Stat,AutoEpbMsgTxt_D_Rq,AwdMde_D_RqBrk,SelDrvMdeMsgTxt_D_Rq,SelDrvMdePos01_B_Avail,SelDrvMdePos02_B_Avail,SelDrvMdePos03_B_Avail,SelDrvMdePos04_B_Avail,SelDrvMdePos05_B_Avail,SelDrvMdePos06_B_Avail,SelDrvMdePos07_B_Avail,SelDrvMdePos08_B_Avail,SelDrvMdePos09_B_Avail,SelDrvMdePos10_B_Avail,SelDrvMdePos11_B_Avail,SelDrvMdePos12_B_Avail,SelDrvMdePt_D_Rq,SelDrvMde_D2_Rq,SelDrvMde_D_Stat
  out_port : Outport
  wires:
  bus_creator/1 -> out_port/1  "SelectDriveModeData"
  ActvDrvMde_D2_Stat/1(out) -> bus_creator/1  "ActvDrvMde_D2_Stat"
  AutoEpbButtnOn_B_Stat/1(out) -> bus_creator/2  "AutoEpbButtnOn_B_Stat"
  AutoEpbDsply_D_Stat/1(out) -> bus_creator/3  "AutoEpbDsply_D_Stat"
  AutoEpbMsgTxt_D_Rq/1(out) -> bus_creator/4  "AutoEpbMsgTxt_D_Rq"
  AwdMde_D_RqBrk/1(out) -> bus_creator/5  "AwdMde_D_RqBrk"
  SelDrvMdeMsgTxt_D_Rq/1(out) -> bus_creator/6  "SelDrvMdeMsgTxt_D_Rq"
  SelDrvMdePos01_B_Avail/1(out) -> bus_creator/7  "SelDrvMdePos01_B_Avail"
  SelDrvMdePos02_B_Avail/1(out) -> bus_creator/8  "SelDrvMdePos02_B_Avail"
  SelDrvMdePos03_B_Avail/1(out) -> bus_creator/9  "SelDrvMdePos03_B_Avail"
  SelDrvMdePos04_B_Avail/1(out) -> bus_creator/10  "SelDrvMdePos04_B_Avail"
  SelDrvMdePos05_B_Avail/1(out) -> bus_creator/11  "SelDrvMdePos05_B_Avail"
  SelDrvMdePos06_B_Avail/1(out) -> bus_creator/12  "SelDrvMdePos06_B_Avail"
  SelDrvMdePos07_B_Avail/1(out) -> bus_creator/13  "SelDrvMdePos07_B_Avail"
  SelDrvMdePos08_B_Avail/1(out) -> bus_creator/14  "SelDrvMdePos08_B_Avail"
  SelDrvMdePos09_B_Avail/1(out) -> bus_creator/15  "SelDrvMdePos09_B_Avail"
  SelDrvMdePos10_B_Avail/1(out) -> bus_creator/16  "SelDrvMdePos10_B_Avail"
  SelDrvMdePos11_B_Avail/1(out) -> bus_creator/17  "SelDrvMdePos11_B_Avail"
  SelDrvMdePos12_B_Avail/1(out) -> bus_creator/18  "SelDrvMdePos12_B_Avail"
  SelDrvMdePt_D_Rq/1(out) -> bus_creator/19  "SelDrvMdePt_D_Rq"
  SelDrvMde_D2_Rq/1(out) -> bus_creator/20  "SelDrvMde_D2_Rq"
  SelDrvMde_D_Stat/1(out) -> bus_creator/21  "SelDrvMde_D_Stat"
  bus_selector/1 -> ActvDrvMde_D2_Stat/1(in)  "<ActvDrvMde_D2_Stat>"
  bus_selector/2 -> AutoEpbButtnOn_B_Stat/1(in)  "<AutoEpbButtnOn_B_Stat>"
  bus_selector/3 -> AutoEpbDsply_D_Stat/1(in)  "<AutoEpbDsply_D_Stat>"
  bus_selector/4 -> AutoEpbMsgTxt_D_Rq/1(in)  "<AutoEpbMsgTxt_D_Rq>"
  bus_selector/5 -> AwdMde_D_RqBrk/1(in)  "<AwdMde_D_RqBrk>"
  bus_selector/6 -> SelDrvMdeMsgTxt_D_Rq/1(in)  "<SelDrvMdeMsgTxt_D_Rq>"
  bus_selector/7 -> SelDrvMdePos01_B_Avail/1(in)  "<SelDrvMdePos01_B_Avail>"
  bus_selector/8 -> SelDrvMdePos02_B_Avail/1(in)  "<SelDrvMdePos02_B_Avail>"
  bus_selector/9 -> SelDrvMdePos03_B_Avail/1(in)  "<SelDrvMdePos03_B_Avail>"
  bus_selector/10 -> SelDrvMdePos04_B_Avail/1(in)  "<SelDrvMdePos04_B_Avail>"
  bus_selector/11 -> SelDrvMdePos05_B_Avail/1(in)  "<SelDrvMdePos05_B_Avail>"
  bus_selector/12 -> SelDrvMdePos06_B_Avail/1(in)  "<SelDrvMdePos06_B_Avail>"
  bus_selector/13 -> SelDrvMdePos07_B_Avail/1(in)  "<SelDrvMdePos07_B_Avail>"
  bus_selector/14 -> SelDrvMdePos08_B_Avail/1(in)  "<SelDrvMdePos08_B_Avail>"
  bus_selector/15 -> SelDrvMdePos09_B_Avail/1(in)  "<SelDrvMdePos09_B_Avail>"
  bus_selector/16 -> SelDrvMdePos10_B_Avail/1(in)  "<SelDrvMdePos10_B_Avail>"
  bus_selector/17 -> SelDrvMdePos11_B_Avail/1(in)  "<SelDrvMdePos11_B_Avail>"
  bus_selector/18 -> SelDrvMdePos12_B_Avail/1(in)  "<SelDrvMdePos12_B_Avail>"
  bus_selector/19 -> SelDrvMdePt_D_Rq/1(in)  "<SelDrvMdePt_D_Rq>"
  bus_selector/20 -> SelDrvMde_D2_Rq/1(in)  "<SelDrvMde_D2_Rq>"
  bus_selector/21 -> SelDrvMde_D_Stat/1(in)  "<SelDrvMde_D_Stat>"
  in/1 -> bus_selector/1

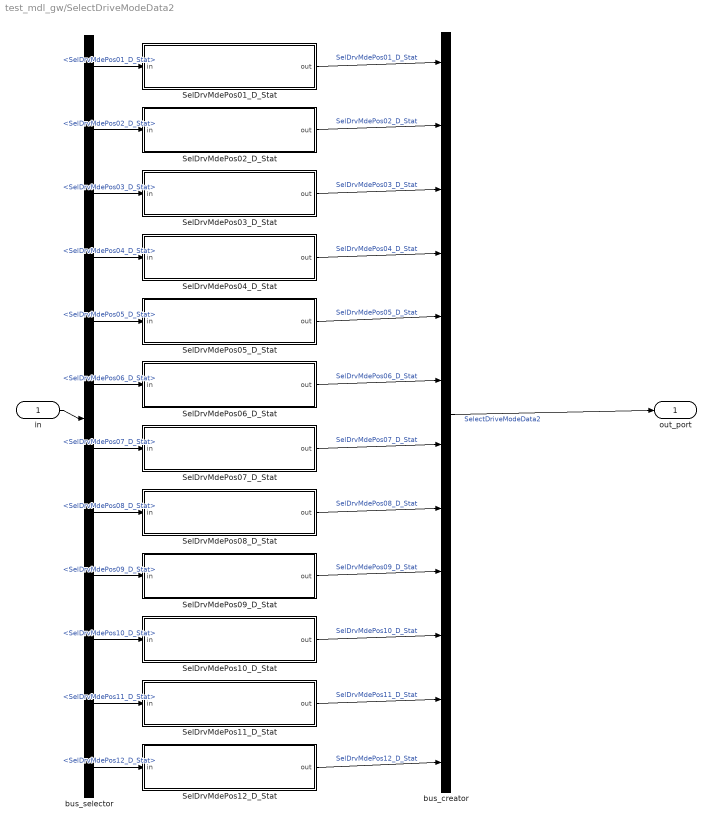
== system test_mdl_gw/SelectDriveModeData2 ==
  in : Inport
  SelDrvMdePos01_D_Stat : Subsystem
  SelDrvMdePos02_D_Stat : Subsystem
  SelDrvMdePos03_D_Stat : Subsystem
  SelDrvMdePos04_D_Stat : Subsystem
  SelDrvMdePos05_D_Stat : Subsystem
  SelDrvMdePos06_D_Stat : Subsystem
  SelDrvMdePos07_D_Stat : Subsystem
  SelDrvMdePos08_D_Stat : Subsystem
  SelDrvMdePos09_D_Stat : Subsystem
  SelDrvMdePos10_D_Stat : Subsystem
  SelDrvMdePos11_D_Stat : Subsystem
  SelDrvMdePos12_D_Stat : Subsystem
  bus_creator : BusCreator  Inputs=12
  bus_selector : BusSelector  OutputSignals=SelDrvMdePos01_D_Stat,SelDrvMdePos02_D_Stat,SelDrvMdePos03_D_Stat,SelDrvMdePos04_D_Stat,SelDrvMdePos05_D_Stat,SelDrvMdePos06_D_Stat,SelDrvMdePos07_D_Stat,SelDrvMdePos08_D_Stat,SelDrvMdePos09_D_Stat,SelDrvMdePos10_D_Stat,SelDrvMdePos11_D_Stat,SelDrvMdePos12_D_Stat
  out_port : Outport
  wires:
  bus_creator/1 -> out_port/1  "SelectDriveModeData2"
  SelDrvMdePos01_D_Stat/1(out) -> bus_creator/1  "SelDrvMdePos01_D_Stat"
  SelDrvMdePos02_D_Stat/1(out) -> bus_creator/2  "SelDrvMdePos02_D_Stat"
  SelDrvMdePos03_D_Stat/1(out) -> bus_creator/3  "SelDrvMdePos03_D_Stat"
  SelDrvMdePos04_D_Stat/1(out) -> bus_creator/4  "SelDrvMdePos04_D_Stat"
  SelDrvMdePos05_D_Stat/1(out) -> bus_creator/5  "SelDrvMdePos05_D_Stat"
  SelDrvMdePos06_D_Stat/1(out) -> bus_creator/6  "SelDrvMdePos06_D_Stat"
  SelDrvMdePos07_D_Stat/1(out) -> bus_creator/7  "SelDrvMdePos07_D_Stat"
  SelDrvMdePos08_D_Stat/1(out) -> bus_creator/8  "SelDrvMdePos08_D_Stat"
  SelDrvMdePos09_D_Stat/1(out) -> bus_creator/9  "SelDrvMdePos09_D_Stat"
  SelDrvMdePos10_D_Stat/1(out) -> bus_creator/10  "SelDrvMdePos10_D_Stat"
  SelDrvMdePos11_D_Stat/1(out) -> bus_creator/11  "SelDrvMdePos11_D_Stat"
  SelDrvMdePos12_D_Stat/1(out) -> bus_creator/12  "SelDrvMdePos12_D_Stat"
  bus_selector/1 -> SelDrvMdePos01_D_Stat/1(in)  "<SelDrvMdePos01_D_Stat>"
  bus_selector/2 -> SelDrvMdePos02_D_Stat/1(in)  "<SelDrvMdePos02_D_Stat>"
  bus_selector/3 -> SelDrvMdePos03_D_Stat/1(in)  "<SelDrvMdePos03_D_Stat>"
  bus_selector/4 -> SelDrvMdePos04_D_Stat/1(in)  "<SelDrvMdePos04_D_Stat>"
  bus_selector/5 -> SelDrvMdePos05_D_Stat/1(in)  "<SelDrvMdePos05_D_Stat>"
  bus_selector/6 -> SelDrvMdePos06_D_Stat/1(in)  "<SelDrvMdePos06_D_Stat>"
  bus_selector/7 -> SelDrvMdePos07_D_Stat/1(in)  "<SelDrvMdePos07_D_Stat>"
  bus_selector/8 -> SelDrvMdePos08_D_Stat/1(in)  "<SelDrvMdePos08_D_Stat>"
  bus_selector/9 -> SelDrvMdePos09_D_Stat/1(in)  "<SelDrvMdePos09_D_Stat>"
  bus_selector/10 -> SelDrvMdePos10_D_Stat/1(in)  "<SelDrvMdePos10_D_Stat>"
  bus_selector/11 -> SelDrvMdePos11_D_Stat/1(in)  "<SelDrvMdePos11_D_Stat>"
  bus_selector/12 -> SelDrvMdePos12_D_Stat/1(in)  "<SelDrvMdePos12_D_Stat>"
  in/1 -> bus_selector/1

== system test_mdl_gw/TesterPhysicalResABS ==
  in : Inport
  TesterPhysicalResABS : Subsystem
  bus_creator : BusCreator  Inputs=1
  bus_selector : BusSelector  OutputSignals=TesterPhysicalResABS
  out_port : Outport
  wires:
  bus_creator/1 -> out_port/1  "TesterPhysicalResABS"
  TesterPhysicalResABS/1(out) -> bus_creator/1  "TesterPhysicalResABS"
  bus_selector/1 -> TesterPhysicalResABS/1(in)  "<TesterPhysicalResABS>"
  in/1 -> bus_selector/1

== system test_mdl_gw/TrailerBrakeData ==
  in : Inport
  TrlrBrk_Pc_Rq : Subsystem
  VehPtch_An_Dsply : Subsystem
  VehRol_An_Dsply : Subsystem
  bus_creator : BusCreator  Inputs=3
  bus_selector : BusSelector  OutputSignals=TrlrBrk_Pc_Rq,VehPtch_An_Dsply,VehRol_An_Dsply
  out_port : Outport
  wires:
  bus_creator/1 -> out_port/1  "TrailerBrakeData"
  TrlrBrk_Pc_Rq/1(out) -> bus_creator/1  "TrlrBrk_Pc_Rq"
  VehPtch_An_Dsply/1(out) -> bus_creator/2  "VehPtch_An_Dsply"
  VehRol_An_Dsply/1(out) -> bus_creator/3  "VehRol_An_Dsply"
  bus_selector/1 -> TrlrBrk_Pc_Rq/1(in)  "<TrlrBrk_Pc_Rq>"
  bus_selector/2 -> VehPtch_An_Dsply/1(in)  "<VehPtch_An_Dsply>"
  bus_selector/3 -> VehRol_An_Dsply/1(in)  "<VehRol_An_Dsply>"
  in/1 -> bus_selector/1

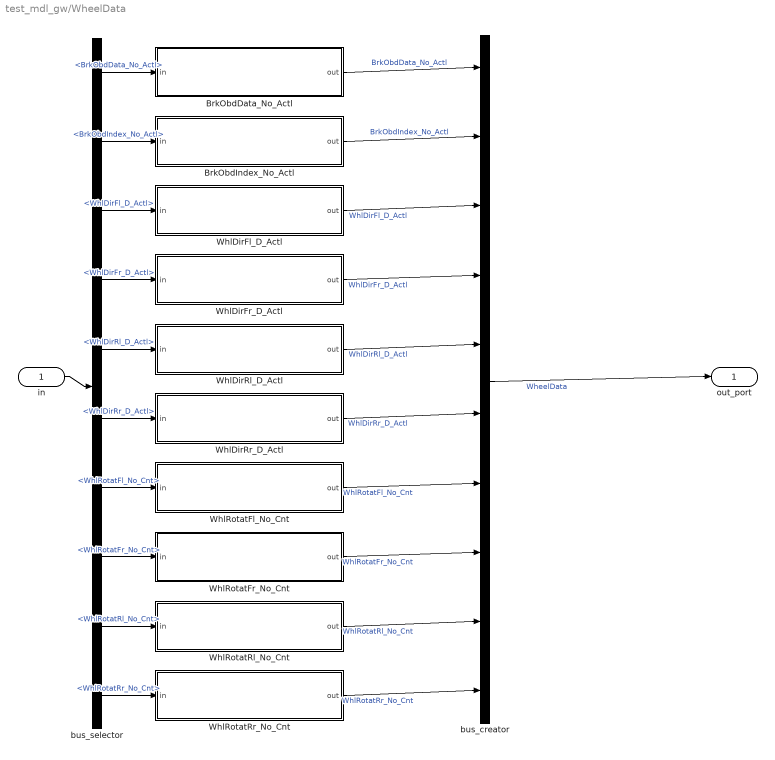
== system test_mdl_gw/WheelData ==
  in : Inport
  BrkObdData_No_Actl : Subsystem
  BrkObdIndex_No_Actl : Subsystem
  WhlDirFl_D_Actl : Subsystem
  WhlDirFr_D_Actl : Subsystem
  WhlDirRl_D_Actl : Subsystem
  WhlDirRr_D_Actl : Subsystem
  WhlRotatFl_No_Cnt : Subsystem
  WhlRotatFr_No_Cnt : Subsystem
  WhlRotatRl_No_Cnt : Subsystem
  WhlRotatRr_No_Cnt : Subsystem
  bus_creator : BusCreator  Inputs=10
  bus_selector : BusSelector  OutputSignals=BrkObdData_No_Actl,BrkObdIndex_No_Actl,WhlDirFl_D_Actl,WhlDirFr_D_Actl,WhlDirRl_D_Actl,WhlDirRr_D_Actl,WhlRotatFl_No_Cnt,WhlRotatFr_No_Cnt,WhlRotatRl_No_Cnt,WhlRotatRr_No_Cnt
  out_port : Outport
  wires:
  bus_creator/1 -> out_port/1  "WheelData"
  BrkObdData_No_Actl/1(out) -> bus_creator/1  "BrkObdData_No_Actl"
  BrkObdIndex_No_Actl/1(out) -> bus_creator/2  "BrkObdIndex_No_Actl"
  WhlDirFl_D_Actl/1(out) -> bus_creator/3  "WhlDirFl_D_Actl"
  WhlDirFr_D_Actl/1(out) -> bus_creator/4  "WhlDirFr_D_Actl"
  WhlDirRl_D_Actl/1(out) -> bus_creator/5  "WhlDirRl_D_Actl"
  WhlDirRr_D_Actl/1(out) -> bus_creator/6  "WhlDirRr_D_Actl"
  WhlRotatFl_No_Cnt/1(out) -> bus_creator/7  "WhlRotatFl_No_Cnt"
  WhlRotatFr_No_Cnt/1(out) -> bus_creator/8  "WhlRotatFr_No_Cnt"
  WhlRotatRl_No_Cnt/1(out) -> bus_creator/9  "WhlRotatRl_No_Cnt"
  WhlRotatRr_No_Cnt/1(out) -> bus_creator/10  "WhlRotatRr_No_Cnt"
  bus_selector/1 -> BrkObdData_No_Actl/1(in)  "<BrkObdData_No_Actl>"
  bus_selector/2 -> BrkObdIndex_No_Actl/1(in)  "<BrkObdIndex_No_Actl>"
  bus_selector/3 -> WhlDirFl_D_Actl/1(in)  "<WhlDirFl_D_Actl>"
  bus_selector/4 -> WhlDirFr_D_Actl/1(in)  "<WhlDirFr_D_Actl>"
  bus_selector/5 -> WhlDirRl_D_Actl/1(in)  "<WhlDirRl_D_Actl>"
  bus_selector/6 -> WhlDirRr_D_Actl/1(in)  "<WhlDirRr_D_Actl>"
  bus_selector/7 -> WhlRotatFl_No_Cnt/1(in)  "<WhlRotatFl_No_Cnt>"
  bus_selector/8 -> WhlRotatFr_No_Cnt/1(in)  "<WhlRotatFr_No_Cnt>"
  bus_selector/9 -> WhlRotatRl_No_Cnt/1(in)  "<WhlRotatRl_No_Cnt>"
  bus_selector/10 -> WhlRotatRr_No_Cnt/1(in)  "<WhlRotatRr_No_Cnt>"
  in/1 -> bus_selector/1

== system test_mdl_gw/WheelSpeed ==
  in : Inport
  WhlFl_W_Meas : Subsystem
  WhlFr_W_Meas : Subsystem
  WhlRl_W_Meas : Subsystem
  WhlRr_W_Meas : Subsystem
  bus_creator : BusCreator  Inputs=4
  bus_selector : BusSelector  OutputSignals=WhlFl_W_Meas,WhlFr_W_Meas,WhlRl_W_Meas,WhlRr_W_Meas
  out_port : Outport
  wires:
  bus_creator/1 -> out_port/1  "WheelSpeed"
  WhlFl_W_Meas/1(out) -> bus_creator/1  "WhlFl_W_Meas"
  WhlFr_W_Meas/1(out) -> bus_creator/2  "WhlFr_W_Meas"
  WhlRl_W_Meas/1(out) -> bus_creator/3  "WhlRl_W_Meas"
  WhlRr_W_Meas/1(out) -> bus_creator/4  "WhlRr_W_Meas"
  bus_selector/1 -> WhlFl_W_Meas/1(in)  "<WhlFl_W_Meas>"
  bus_selector/2 -> WhlFr_W_Meas/1(in)  "<WhlFr_W_Meas>"
  bus_selector/3 -> WhlRl_W_Meas/1(in)  "<WhlRl_W_Meas>"
  bus_selector/4 -> WhlRr_W_Meas/1(in)  "<WhlRr_W_Meas>"
  in/1 -> bus_selector/1

== system test_mdl_gw/ABS_AutoSar_NetworkMgt/ABS_AutoSarNMControl ==
  in : Inport
  out : Outport
  wires:
  in/1 -> out/1

== system test_mdl_gw/ABS_AutoSar_NetworkMgt/ABS_AutoSarNMNodeId ==
  in : Inport
  out : Outport
  wires:
  in/1 -> out/1

== system test_mdl_gw/ABS_AutoSar_NetworkMgt/ABS_AutoSarNMReserved1 ==
  in : Inport
  out : Outport
  wires:
  in/1 -> out/1

== system test_mdl_gw/ABS_AutoSar_NetworkMgt/ABS_AutoSarNMReserved2 ==
  in : Inport
  out : Outport
  wires:
  in/1 -> out/1

== system test_mdl_gw/ABS_AutoSar_NetworkMgt/ABS_AutoSarNMReserved3 ==
  in : Inport
  out : Outport
  wires:
  in/1 -> out/1

== system test_mdl_gw/ABS_AutoSar_NetworkMgt/ABS_AutoSarNMReserved4 ==
  in : Inport
  out : Outport
  wires:
  in/1 -> out/1

== system test_mdl_gw/ABS_AutoSar_NetworkMgt/ABS_GWNMProxy ==
  in : Inport
  out : Outport
  wires:
  in/1 -> out/1

== system test_mdl_gw/ABS_AutoSar_NetworkMgt/ABS_GWOnBoardTester ==
  in : Inport
  out : Outport
  wires:
  in/1 -> out/1

== system test_mdl_gw/ABS_AutoSar_NetworkMgt/a ==
  Out1 : Outport

== system test_mdl_gw/ABS_AutoSar_NetworkMgt/b ==
  Out1 : Outport

== system test_mdl_gw/ABS_BrkBst_Data/BrkBstrVac_P_Actl ==
  in : Inport
  out : Outport
  wires:
  in/1 -> out/1

== system test_mdl_gw/ABS_BrkBst_Data/BrkHold_D_Stat ==
  in : Inport
  out : Outport
  wires:
  in/1 -> out/1

== system test_mdl_gw/ABS_BrkBst_Data/BrkTotTqRqDrv_No_Cnt ==
  in : Inport
  out : Outport
  wires:
  in/1 -> out/1

== system test_mdl_gw/ABS_BrkBst_Data/BrkTotTqRqDrv_No_Cs ==
  in : Inport
  out : Outport
  wires:
  in/1 -> out/1

== system test_mdl_gw/ABS_BrkBst_Data/BrkTot_Tq_RqDrv ==
  in : Inport
  out : Outport
  wires:
  in/1 -> out/1

== system test_mdl_gw/ABS_BrkBst_Data/HsaStat_D_Dsply ==
  in : Inport
  out : Outport
  wires:
  in/1 -> out/1

== system test_mdl_gw/ABS_BrkBst_Data/HsaTrnAout_Tq_Rq ==
  in : Inport
  out : Outport
  wires:
  in/1 -> out/1

== system test_mdl_gw/ABS_BrkBst_Data/YawStabilityIndex ==
  in : Inport
  out : Outport
  wires:
  in/1 -> out/1

== system test_mdl_gw/ABS_Rapid_Data_Response_1/UUDTABSResponse1 ==
  in : Inport
  out : Outport
  wires:
  in/1 -> out/1

== system test_mdl_gw/ABS_Rapid_Data_Response_2/UUDTABSResponse2 ==
  in : Inport
  out : Outport
  wires:
  in/1 -> out/1

== system test_mdl_gw/ActiveFronSteering_Req/SteWhlBrkAnRq_No_Cnt ==
  in : Inport
  out : Outport
  wires:
  in/1 -> out/1

== system test_mdl_gw/ActiveFronSteering_Req/SteWhlBrkAnRq_No_Cs ==
  in : Inport
  out : Outport
  wires:
  in/1 -> out/1

== system test_mdl_gw/ActiveFronSteering_Req/SteWhlBrkOffst_An_Rq ==
  in : Inport
  out : Outport
  wires:
  in/1 -> out/1

== system test_mdl_gw/BrakeSnData_3/VehLatComp_A_Actl ==
  in : Inport
  out : Outport
  wires:
  in/1 -> out/1

== system test_mdl_gw/BrakeSnData_3/VehLongComp_A_Actl ==
  in : Inport
  out : Outport
  wires:
  in/1 -> out/1

== system test_mdl_gw/BrakeSnData_3/VehOverGnd_V_Est ==
  in : Inport
  out : Outport
  wires:
  in/1 -> out/1

== system test_mdl_gw/BrakeSnData_3/VehTrvlDir_D_Stat ==
  in : Inport
  out : Outport
  wires:
  in/1 -> out/1

== system test_mdl_gw/BrakeSnData_3/VehYawComp_W_Actl ==
  in : Inport
  out : Outport
  wires:
  in/1 -> out/1

== system test_mdl_gw/BrakeSnData_4/BrkTotTqRqArb_No_Cnt ==
  in : Inport
  out : Outport
  wires:
  in/1 -> out/1

== system test_mdl_gw/BrakeSnData_4/BrkTotTqRqArb_No_Cs ==
  in : Inport
  out : Outport
  wires:
  in/1 -> out/1

== system test_mdl_gw/BrakeSnData_4/BrkTot_Tq_Actl ==
  in : Inport
  out : Outport
  wires:
  in/1 -> out/1

== system test_mdl_gw/BrakeSnData_4/BrkTot_Tq_RqArb ==
  in : Inport
  out : Outport
  wires:
  in/1 -> out/1

== system test_mdl_gw/BrakeSnData_4/HsaStat_D_Actl ==
  in : Inport
  out : Outport
  wires:
  in/1 -> out/1

== system test_mdl_gw/BrakeSnData_4/VehRolComp_W_Actl ==
  in : Inport
  out : Outport
  wires:
  in/1 -> out/1

== system test_mdl_gw/BrakeSnData_4/VehVertComp_A_Actl ==
  in : Inport
  out : Outport
  wires:
  in/1 -> out/1

== system test_mdl_gw/BrakeSnData_5/AwdLck_Tq_RqMn ==
  in : Inport
  out : Outport
  wires:
  in/1 -> out/1

== system test_mdl_gw/BrakeSnData_5/AwdLck_Tq_RqMx ==
  in : Inport
  out : Outport
  wires:
  in/1 -> out/1

== system test_mdl_gw/BrakeSnData_5/BrkCtrFnd_B_Stat ==
  in : Inport
  out : Outport
  wires:
  in/1 -> out/1

== system test_mdl_gw/BrakeSnData_5/DrvSte_D_Stat ==
  in : Inport
  out : Outport
  wires:
  in/1 -> out/1

== system test_mdl_gw/BrakeSnData_5/DrvSte_Tq_Rq ==
  in : Inport
  out : Outport
  wires:
  in/1 -> out/1

== system test_mdl_gw/BrakeSnData_5/EmgcyBrkLamp_D_Rq ==
  in : Inport
  out : Outport
  wires:
  in/1 -> out/1

== system test_mdl_gw/BrakeSnData_5/StopLamp_B_RqBrk ==
  in : Inport
  out : Outport
  wires:
  in/1 -> out/1

== system test_mdl_gw/BrakeSnData_6/StePinOffst_An_Est ==
  in : Inport
  out : Outport
  wires:
  in/1 -> out/1

== system test_mdl_gw/BrakeSnData_6/StePinOffst_D_Stat ==
  in : Inport
  out : Outport
  wires:
  in/1 -> out/1

== system test_mdl_gw/BrakeSnData_6/StePinOffst_No_Cnt ==
  in : Inport
  out : Outport
  wires:
  in/1 -> out/1

== system test_mdl_gw/BrakeSnData_6/StePinOffst_No_Cs ==
  in : Inport
  out : Outport
  wires:
  in/1 -> out/1

== system test_mdl_gw/BrakeSysFeatures/BrkFluidLvl_D_Stat ==
  in : Inport
  out : Outport
  wires:
  in/1 -> out/1

== system test_mdl_gw/BrakeSysFeatures/LsmcBrkDecel_D_Stat ==
  in : Inport
  out : Outport
  wires:
  in/1 -> out/1

== system test_mdl_gw/BrakeSysFeatures/VehStab_D_Stat ==
  in : Inport
  out : Outport
  wires:
  in/1 -> out/1

== system test_mdl_gw/BrakeSysFeatures/VehVActlBrk_D_Qf ==
  in : Inport
  out : Outport
  wires:
  in/1 -> out/1

== system test_mdl_gw/BrakeSysFeatures/VehVActlBrk_No_Cnt ==
  in : Inport
  out : Outport
  wires:
  in/1 -> out/1

== system test_mdl_gw/BrakeSysFeatures/VehVActlBrk_No_Cs ==
  in : Inport
  out : Outport
  wires:
  in/1 -> out/1

== system test_mdl_gw/BrakeSysFeatures/VehYawLin_W_Rq ==
  in : Inport
  out : Outport
  wires:
  in/1 -> out/1

== system test_mdl_gw/BrakeSysFeatures/VehYawNonLin_W_Rq ==
  in : Inport
  out : Outport
  wires:
  in/1 -> out/1

== system test_mdl_gw/BrakeSysFeatures/Veh_V_ActlBrk ==
  in : Inport
  out : Outport
  wires:
  in/1 -> out/1

== system test_mdl_gw/BrakeSysFeatures_2/Abs_B_Falt ==
  in : Inport
  out : Outport
  wires:
  in/1 -> out/1

== system test_mdl_gw/BrakeSysFeatures_2/BpedMove_D_Actl ==
  in : Inport
  out : Outport
  wires:
  in/1 -> out/1

== system test_mdl_gw/BrakeSysFeatures_2/BpedMove_No_Cnt ==
  in : Inport
  out : Outport
  wires:
  in/1 -> out/1

== system test_mdl_gw/BrakeSysFeatures_2/BrkBstrVac_B_Rq ==
  in : Inport
  out : Outport
  wires:
  in/1 -> out/1

== system test_mdl_gw/BrakeSysFeatures_2/BrkLamp_B_Rq ==
  in : Inport
  out : Outport
  wires:
  in/1 -> out/1

== system test_mdl_gw/BrakeSysFeatures_2/ChimeBrk_B_Rq ==
  in : Inport
  out : Outport
  wires:
  in/1 -> out/1

== system test_mdl_gw/BrakeSysFeatures_2/DrvAntiLckLamp_D_Rq ==
  in : Inport
  out : Outport
  wires:
  in/1 -> out/1

== system test_mdl_gw/BrakeSysFeatures_2/DrvHdcLampInfo_D_Rq ==
  in : Inport
  out : Outport
  wires:
  in/1 -> out/1

== system test_mdl_gw/BrakeSysFeatures_2/DrvHdcMsg_D_Rq ==
  in : Inport
  out : Outport
  wires:
  in/1 -> out/1

== system test_mdl_gw/BrakeSysFeatures_2/DrvHdcWarnInfo_D_Rq ==
  in : Inport
  out : Outport
  wires:
  in/1 -> out/1

== system test_mdl_gw/BrakeSysFeatures_2/DrvSlipCtlLamp_D_Rq ==
  in : Inport
  out : Outport
  wires:
  in/1 -> out/1

== system test_mdl_gw/BrakeSysFeatures_2/DrvSlipCtlMde_D_Ind ==
  in : Inport
  out : Outport
  wires:
  in/1 -> out/1

== system test_mdl_gw/BrakeSysFeatures_2/HILL_DESC_MC ==
  in : Inport
  out : Outport
  wires:
  in/1 -> out/1

== system test_mdl_gw/BrakeSysFeatures_2/HdcMde_D_Actl ==
  in : Inport
  out : Outport
  wires:
  in/1 -> out/1

== system test_mdl_gw/BrakeSysFeatures_2/HsaMde_D_Mem ==
  in : Inport
  out : Outport
  wires:
  in/1 -> out/1

== system test_mdl_gw/BrakeSysFeatures_2/RearDiffElckrOpen_B_Rq ==
  in : Inport
  out : Outport
  wires:
  in/1 -> out/1

== system test_mdl_gw/BrakeSysFeatures_2/RearDiffLck_Tq2_RqMx ==
  in : Inport
  out : Outport
  wires:
  in/1 -> out/1

== system test_mdl_gw/BrakeSysFeatures_2/StabCtlBrk_B_Avail ==
  in : Inport
  out : Outport
  wires:
  in/1 -> out/1

== system test_mdl_gw/BrakeSysFeatures_2/TCMode ==
  in : Inport
  out : Outport
  wires:
  in/1 -> out/1

== system test_mdl_gw/BrakeSysFeatures_2/TRLR_SWAY_CONFIG_STAT ==
  in : Inport
  out : Outport
  wires:
  in/1 -> out/1
